simulink model "ADU_Integration_Y2016_simulation"  (R2016b)
settings: Solver=FixedStepDiscrete  StartTime=240  StopTime=300  FixedStep=0.01  RelTol=1e-3  EnableMultiTasking=on
PostLoadFcn:
  | , if any(exist('dsrtsu_mdlpostloadfcn', 'file') == [2, 3, 6]), try dsrtsu_mdlpostloadfcn('Execute', bdroot); catch fprintf('Error in PostLoadFcn (dsrtsu_mdlpostloadfcn) for model "%s":\n %s\n', bdroot, lasterr); end, end,
InitFcn:
  | load 'data/chi2_dat';
  | load 'data/innerLine_struct';
  | load 'data/middleLine_struct';
  | load 'data/outerLine_struct';
  | load 'data/innerLine';
  | load 'data/middleLine';
  | load 'data/outerLine';
  | load 'data/landmarks_patac_schimmel_ccw';
  | load 'data/patac_navi_array';
  | load 'data/sensor';
  | load 'data/map_struct';
  | addpath map_src
  | Integration_Parameter;
  | load 'TestData_001';
values from neighbouring files (symbols this model uses):
  TestData_001 =     [TestData_001.mat]
undefined symbols (not defined in the file or in its folder): a, chi2_dat, innerLine, landmarks_patac_schimmel_ccw, middleLine, outerLine, patac_navi_array, StartNum
libraries: simulink x36, rtican x1
(part 4 of 20)

== system ADU_Integration_Y2016_simulation/LogData/Sensor_ESR/Data_13 ==
  1-D Lookup Table1 : Lookup_n-D  NumberOfTableDimensions=1  BreakpointsForDimension1=TestData_001.X.Data  Table=TestData_001.Y(206+4*a).Data  RndMeth=Simplest  InputSameDT=on
  1-D Lookup Table2 : Lookup_n-D  NumberOfTableDimensions=1  BreakpointsForDimension1=TestData_001.X.Data  Table=TestData_001.Y(205+4*a).Data  RndMeth=Simplest  InputSameDT=on
  1-D Lookup Table3 : Lookup_n-D  NumberOfTableDimensions=1  BreakpointsForDimension1=TestData_001.X.Data  Table=TestData_001.Y(207+4*a).Data  RndMeth=Simplest  InputSameDT=on
  1-D Lookup Table4 : Lookup_n-D  NumberOfTableDimensions=1  BreakpointsForDimension1=TestData_001.X.Data  Table=TestData_001.Y(208+4*a).Data  RndMeth=Simplest  InputSameDT=on
  Mux5 : Mux
  Quantizer9 : Quantizer  QuantizationInterval=1
  Out1 : Outport
  wires:
  Mux5/1 -> Out1/1
  [Clock] -> 1-D Lookup Table2/1, 1-D Lookup Table4/1, 1-D Lookup Table3/1, 1-D Lookup Table1/1
  1-D Lookup Table4/1 -> Mux5/4
  Quantizer9/1 -> Mux5/1
  1-D Lookup Table2/1 -> Quantizer9/1
  1-D Lookup Table1/1 -> Mux5/2  "Data"
  1-D Lookup Table3/1 -> Mux5/3

== system ADU_Integration_Y2016_simulation/LogData/Sensor_ESR/Data_14 ==
  1-D Lookup Table1 : Lookup_n-D  NumberOfTableDimensions=1  BreakpointsForDimension1=TestData_001.X.Data  Table=TestData_001.Y(206+4*a).Data  RndMeth=Simplest  InputSameDT=on
  1-D Lookup Table2 : Lookup_n-D  NumberOfTableDimensions=1  BreakpointsForDimension1=TestData_001.X.Data  Table=TestData_001.Y(205+4*a).Data  RndMeth=Simplest  InputSameDT=on
  1-D Lookup Table3 : Lookup_n-D  NumberOfTableDimensions=1  BreakpointsForDimension1=TestData_001.X.Data  Table=TestData_001.Y(207+4*a).Data  RndMeth=Simplest  InputSameDT=on
  1-D Lookup Table4 : Lookup_n-D  NumberOfTableDimensions=1  BreakpointsForDimension1=TestData_001.X.Data  Table=TestData_001.Y(208+4*a).Data  RndMeth=Simplest  InputSameDT=on
  Mux5 : Mux
  Quantizer9 : Quantizer  QuantizationInterval=1
  Out1 : Outport
  wires:
  1-D Lookup Table3/1 -> Mux5/3
  1-D Lookup Table1/1 -> Mux5/2  "Data"
  1-D Lookup Table2/1 -> Quantizer9/1
  Quantizer9/1 -> Mux5/1
  1-D Lookup Table4/1 -> Mux5/4
  [Clock] -> 1-D Lookup Table1/1, 1-D Lookup Table3/1, 1-D Lookup Table4/1, 1-D Lookup Table2/1
  Mux5/1 -> Out1/1

== system ADU_Integration_Y2016_simulation/LogData/Sensor_ESR/Data_15 ==
  1-D Lookup Table1 : Lookup_n-D  NumberOfTableDimensions=1  BreakpointsForDimension1=TestData_001.X.Data  Table=TestData_001.Y(206+4*a).Data  RndMeth=Simplest  InputSameDT=on
  1-D Lookup Table2 : Lookup_n-D  NumberOfTableDimensions=1  BreakpointsForDimension1=TestData_001.X.Data  Table=TestData_001.Y(205+4*a).Data  RndMeth=Simplest  InputSameDT=on
  1-D Lookup Table3 : Lookup_n-D  NumberOfTableDimensions=1  BreakpointsForDimension1=TestData_001.X.Data  Table=TestData_001.Y(207+4*a).Data  RndMeth=Simplest  InputSameDT=on
  1-D Lookup Table4 : Lookup_n-D  NumberOfTableDimensions=1  BreakpointsForDimension1=TestData_001.X.Data  Table=TestData_001.Y(208+4*a).Data  RndMeth=Simplest  InputSameDT=on
  Mux5 : Mux
  Quantizer9 : Quantizer  QuantizationInterval=1
  Out1 : Outport
  wires:
  Mux5/1 -> Out1/1
  [Clock] -> 1-D Lookup Table2/1, 1-D Lookup Table4/1, 1-D Lookup Table3/1, 1-D Lookup Table1/1
  1-D Lookup Table4/1 -> Mux5/4
  Quantizer9/1 -> Mux5/1
  1-D Lookup Table2/1 -> Quantizer9/1
  1-D Lookup Table1/1 -> Mux5/2  "Data"
  1-D Lookup Table3/1 -> Mux5/3

== system ADU_Integration_Y2016_simulation/LogData/Sensor_ESR/Data_16 ==
  1-D Lookup Table1 : Lookup_n-D  NumberOfTableDimensions=1  BreakpointsForDimension1=TestData_001.X.Data  Table=TestData_001.Y(206+4*a).Data  RndMeth=Simplest  InputSameDT=on
  1-D Lookup Table2 : Lookup_n-D  NumberOfTableDimensions=1  BreakpointsForDimension1=TestData_001.X.Data  Table=TestData_001.Y(205+4*a).Data  RndMeth=Simplest  InputSameDT=on
  1-D Lookup Table3 : Lookup_n-D  NumberOfTableDimensions=1  BreakpointsForDimension1=TestData_001.X.Data  Table=TestData_001.Y(207+4*a).Data  RndMeth=Simplest  InputSameDT=on
  1-D Lookup Table4 : Lookup_n-D  NumberOfTableDimensions=1  BreakpointsForDimension1=TestData_001.X.Data  Table=TestData_001.Y(208+4*a).Data  RndMeth=Simplest  InputSameDT=on
  Mux5 : Mux
  Quantizer9 : Quantizer  QuantizationInterval=1
  Out1 : Outport
  wires:
  1-D Lookup Table3/1 -> Mux5/3
  1-D Lookup Table1/1 -> Mux5/2  "Data"
  1-D Lookup Table2/1 -> Quantizer9/1
  Quantizer9/1 -> Mux5/1
  1-D Lookup Table4/1 -> Mux5/4
  [Clock] -> 1-D Lookup Table1/1, 1-D Lookup Table3/1, 1-D Lookup Table4/1, 1-D Lookup Table2/1
  Mux5/1 -> Out1/1

== system ADU_Integration_Y2016_simulation/LogData/Sensor_ESR/Data_17 ==
  1-D Lookup Table1 : Lookup_n-D  NumberOfTableDimensions=1  BreakpointsForDimension1=TestData_001.X.Data  Table=TestData_001.Y(206+4*a).Data  RndMeth=Simplest  InputSameDT=on
  1-D Lookup Table2 : Lookup_n-D  NumberOfTableDimensions=1  BreakpointsForDimension1=TestData_001.X.Data  Table=TestData_001.Y(205+4*a).Data  RndMeth=Simplest  InputSameDT=on
  1-D Lookup Table3 : Lookup_n-D  NumberOfTableDimensions=1  BreakpointsForDimension1=TestData_001.X.Data  Table=TestData_001.Y(207+4*a).Data  RndMeth=Simplest  InputSameDT=on
  1-D Lookup Table4 : Lookup_n-D  NumberOfTableDimensions=1  BreakpointsForDimension1=TestData_001.X.Data  Table=TestData_001.Y(208+4*a).Data  RndMeth=Simplest  InputSameDT=on
  Mux5 : Mux
  Quantizer9 : Quantizer  QuantizationInterval=1
  Out1 : Outport
  wires:
  Mux5/1 -> Out1/1
  [Clock] -> 1-D Lookup Table2/1, 1-D Lookup Table4/1, 1-D Lookup Table3/1, 1-D Lookup Table1/1
  1-D Lookup Table4/1 -> Mux5/4
  Quantizer9/1 -> Mux5/1
  1-D Lookup Table2/1 -> Quantizer9/1
  1-D Lookup Table1/1 -> Mux5/2  "Data"
  1-D Lookup Table3/1 -> Mux5/3

== system ADU_Integration_Y2016_simulation/LogData/Sensor_ESR/Data_18 ==
  1-D Lookup Table1 : Lookup_n-D  NumberOfTableDimensions=1  BreakpointsForDimension1=TestData_001.X.Data  Table=TestData_001.Y(206+4*a).Data  RndMeth=Simplest  InputSameDT=on
  1-D Lookup Table2 : Lookup_n-D  NumberOfTableDimensions=1  BreakpointsForDimension1=TestData_001.X.Data  Table=TestData_001.Y(205+4*a).Data  RndMeth=Simplest  InputSameDT=on
  1-D Lookup Table3 : Lookup_n-D  NumberOfTableDimensions=1  BreakpointsForDimension1=TestData_001.X.Data  Table=TestData_001.Y(207+4*a).Data  RndMeth=Simplest  InputSameDT=on
  1-D Lookup Table4 : Lookup_n-D  NumberOfTableDimensions=1  BreakpointsForDimension1=TestData_001.X.Data  Table=TestData_001.Y(208+4*a).Data  RndMeth=Simplest  InputSameDT=on
  Mux5 : Mux
  Quantizer9 : Quantizer  QuantizationInterval=1
  Out1 : Outport
  wires:
  1-D Lookup Table3/1 -> Mux5/3
  1-D Lookup Table1/1 -> Mux5/2  "Data"
  1-D Lookup Table2/1 -> Quantizer9/1
  Quantizer9/1 -> Mux5/1
  1-D Lookup Table4/1 -> Mux5/4
  [Clock] -> 1-D Lookup Table1/1, 1-D Lookup Table3/1, 1-D Lookup Table4/1, 1-D Lookup Table2/1
  Mux5/1 -> Out1/1

== system ADU_Integration_Y2016_simulation/LogData/Sensor_ESR/Data_19 ==
  1-D Lookup Table1 : Lookup_n-D  NumberOfTableDimensions=1  BreakpointsForDimension1=TestData_001.X.Data  Table=TestData_001.Y(206+4*a).Data  RndMeth=Simplest  InputSameDT=on
  1-D Lookup Table2 : Lookup_n-D  NumberOfTableDimensions=1  BreakpointsForDimension1=TestData_001.X.Data  Table=TestData_001.Y(205+4*a).Data  RndMeth=Simplest  InputSameDT=on
  1-D Lookup Table3 : Lookup_n-D  NumberOfTableDimensions=1  BreakpointsForDimension1=TestData_001.X.Data  Table=TestData_001.Y(207+4*a).Data  RndMeth=Simplest  InputSameDT=on
  1-D Lookup Table4 : Lookup_n-D  NumberOfTableDimensions=1  BreakpointsForDimension1=TestData_001.X.Data  Table=TestData_001.Y(208+4*a).Data  RndMeth=Simplest  InputSameDT=on
  Mux5 : Mux
  Quantizer9 : Quantizer  QuantizationInterval=1
  Out1 : Outport
  wires:
  Mux5/1 -> Out1/1
  [Clock] -> 1-D Lookup Table2/1, 1-D Lookup Table4/1, 1-D Lookup Table3/1, 1-D Lookup Table1/1
  1-D Lookup Table4/1 -> Mux5/4
  Quantizer9/1 -> Mux5/1
  1-D Lookup Table2/1 -> Quantizer9/1
  1-D Lookup Table1/1 -> Mux5/2  "Data"
  1-D Lookup Table3/1 -> Mux5/3

== system ADU_Integration_Y2016_simulation/LogData/Sensor_ESR/Data_2 ==
  1-D Lookup Table1 : Lookup_n-D  NumberOfTableDimensions=1  BreakpointsForDimension1=TestData_001.X.Data  Table=TestData_001.Y(206+4*a).Data  RndMeth=Simplest  InputSameDT=on
  1-D Lookup Table2 : Lookup_n-D  NumberOfTableDimensions=1  BreakpointsForDimension1=TestData_001.X.Data  Table=TestData_001.Y(205+4*a).Data  RndMeth=Simplest  InputSameDT=on
  1-D Lookup Table3 : Lookup_n-D  NumberOfTableDimensions=1  BreakpointsForDimension1=TestData_001.X.Data  Table=TestData_001.Y(207+4*a).Data  RndMeth=Simplest  InputSameDT=on
  1-D Lookup Table4 : Lookup_n-D  NumberOfTableDimensions=1  BreakpointsForDimension1=TestData_001.X.Data  Table=TestData_001.Y(208+4*a).Data  RndMeth=Simplest  InputSameDT=on
  Mux5 : Mux
  Quantizer9 : Quantizer  QuantizationInterval=1
  Out1 : Outport
  wires:
  1-D Lookup Table3/1 -> Mux5/3
  1-D Lookup Table1/1 -> Mux5/2  "Data"
  1-D Lookup Table2/1 -> Quantizer9/1
  Quantizer9/1 -> Mux5/1
  1-D Lookup Table4/1 -> Mux5/4
  [Clock] -> 1-D Lookup Table1/1, 1-D Lookup Table3/1, 1-D Lookup Table4/1, 1-D Lookup Table2/1
  Mux5/1 -> Out1/1

== system ADU_Integration_Y2016_simulation/LogData/Sensor_ESR/Data_20 ==
  1-D Lookup Table1 : Lookup_n-D  NumberOfTableDimensions=1  BreakpointsForDimension1=TestData_001.X.Data  Table=TestData_001.Y(206+4*a).Data  RndMeth=Simplest  InputSameDT=on
  1-D Lookup Table2 : Lookup_n-D  NumberOfTableDimensions=1  BreakpointsForDimension1=TestData_001.X.Data  Table=TestData_001.Y(205+4*a).Data  RndMeth=Simplest  InputSameDT=on
  1-D Lookup Table3 : Lookup_n-D  NumberOfTableDimensions=1  BreakpointsForDimension1=TestData_001.X.Data  Table=TestData_001.Y(207+4*a).Data  RndMeth=Simplest  InputSameDT=on
  1-D Lookup Table4 : Lookup_n-D  NumberOfTableDimensions=1  BreakpointsForDimension1=TestData_001.X.Data  Table=TestData_001.Y(208+4*a).Data  RndMeth=Simplest  InputSameDT=on
  Mux5 : Mux
  Quantizer9 : Quantizer  QuantizationInterval=1
  Out1 : Outport
  wires:
  1-D Lookup Table3/1 -> Mux5/3
  1-D Lookup Table1/1 -> Mux5/2  "Data"
  1-D Lookup Table2/1 -> Quantizer9/1
  Quantizer9/1 -> Mux5/1
  1-D Lookup Table4/1 -> Mux5/4
  [Clock] -> 1-D Lookup Table1/1, 1-D Lookup Table3/1, 1-D Lookup Table4/1, 1-D Lookup Table2/1
  Mux5/1 -> Out1/1

== system ADU_Integration_Y2016_simulation/LogData/Sensor_ESR/Data_21 ==
  1-D Lookup Table1 : Lookup_n-D  NumberOfTableDimensions=1  BreakpointsForDimension1=TestData_001.X.Data  Table=TestData_001.Y(206+4*a).Data  RndMeth=Simplest  InputSameDT=on
  1-D Lookup Table2 : Lookup_n-D  NumberOfTableDimensions=1  BreakpointsForDimension1=TestData_001.X.Data  Table=TestData_001.Y(205+4*a).Data  RndMeth=Simplest  InputSameDT=on
  1-D Lookup Table3 : Lookup_n-D  NumberOfTableDimensions=1  BreakpointsForDimension1=TestData_001.X.Data  Table=TestData_001.Y(207+4*a).Data  RndMeth=Simplest  InputSameDT=on
  1-D Lookup Table4 : Lookup_n-D  NumberOfTableDimensions=1  BreakpointsForDimension1=TestData_001.X.Data  Table=TestData_001.Y(208+4*a).Data  RndMeth=Simplest  InputSameDT=on
  Mux5 : Mux
  Quantizer9 : Quantizer  QuantizationInterval=1
  Out1 : Outport
  wires:
  Mux5/1 -> Out1/1
  [Clock] -> 1-D Lookup Table2/1, 1-D Lookup Table4/1, 1-D Lookup Table3/1, 1-D Lookup Table1/1
  1-D Lookup Table4/1 -> Mux5/4
  Quantizer9/1 -> Mux5/1
  1-D Lookup Table2/1 -> Quantizer9/1
  1-D Lookup Table1/1 -> Mux5/2  "Data"
  1-D Lookup Table3/1 -> Mux5/3

== system ADU_Integration_Y2016_simulation/LogData/Sensor_ESR/Data_22 ==
  1-D Lookup Table1 : Lookup_n-D  NumberOfTableDimensions=1  BreakpointsForDimension1=TestData_001.X.Data  Table=TestData_001.Y(206+4*a).Data  RndMeth=Simplest  InputSameDT=on
  1-D Lookup Table2 : Lookup_n-D  NumberOfTableDimensions=1  BreakpointsForDimension1=TestData_001.X.Data  Table=TestData_001.Y(205+4*a).Data  RndMeth=Simplest  InputSameDT=on
  1-D Lookup Table3 : Lookup_n-D  NumberOfTableDimensions=1  BreakpointsForDimension1=TestData_001.X.Data  Table=TestData_001.Y(207+4*a).Data  RndMeth=Simplest  InputSameDT=on
  1-D Lookup Table4 : Lookup_n-D  NumberOfTableDimensions=1  BreakpointsForDimension1=TestData_001.X.Data  Table=TestData_001.Y(208+4*a).Data  RndMeth=Simplest  InputSameDT=on
  Mux5 : Mux
  Quantizer9 : Quantizer  QuantizationInterval=1
  Out1 : Outport
  wires:
  1-D Lookup Table3/1 -> Mux5/3
  1-D Lookup Table1/1 -> Mux5/2  "Data"
  1-D Lookup Table2/1 -> Quantizer9/1
  Quantizer9/1 -> Mux5/1
  1-D Lookup Table4/1 -> Mux5/4
  [Clock] -> 1-D Lookup Table1/1, 1-D Lookup Table3/1, 1-D Lookup Table4/1, 1-D Lookup Table2/1
  Mux5/1 -> Out1/1

== system ADU_Integration_Y2016_simulation/LogData/Sensor_ESR/Data_23 ==
  1-D Lookup Table1 : Lookup_n-D  NumberOfTableDimensions=1  BreakpointsForDimension1=TestData_001.X.Data  Table=TestData_001.Y(206+4*a).Data  RndMeth=Simplest  InputSameDT=on
  1-D Lookup Table2 : Lookup_n-D  NumberOfTableDimensions=1  BreakpointsForDimension1=TestData_001.X.Data  Table=TestData_001.Y(205+4*a).Data  RndMeth=Simplest  InputSameDT=on
  1-D Lookup Table3 : Lookup_n-D  NumberOfTableDimensions=1  BreakpointsForDimension1=TestData_001.X.Data  Table=TestData_001.Y(207+4*a).Data  RndMeth=Simplest  InputSameDT=on
  1-D Lookup Table4 : Lookup_n-D  NumberOfTableDimensions=1  BreakpointsForDimension1=TestData_001.X.Data  Table=TestData_001.Y(208+4*a).Data  RndMeth=Simplest  InputSameDT=on
  Mux5 : Mux
  Quantizer9 : Quantizer  QuantizationInterval=1
  Out1 : Outport
  wires:
  Mux5/1 -> Out1/1
  [Clock] -> 1-D Lookup Table2/1, 1-D Lookup Table4/1, 1-D Lookup Table3/1, 1-D Lookup Table1/1
  1-D Lookup Table4/1 -> Mux5/4
  Quantizer9/1 -> Mux5/1
  1-D Lookup Table2/1 -> Quantizer9/1
  1-D Lookup Table1/1 -> Mux5/2  "Data"
  1-D Lookup Table3/1 -> Mux5/3

== system ADU_Integration_Y2016_simulation/LogData/Sensor_ESR/Data_24 ==
  1-D Lookup Table1 : Lookup_n-D  NumberOfTableDimensions=1  BreakpointsForDimension1=TestData_001.X.Data  Table=TestData_001.Y(206+4*a).Data  RndMeth=Simplest  InputSameDT=on
  1-D Lookup Table2 : Lookup_n-D  NumberOfTableDimensions=1  BreakpointsForDimension1=TestData_001.X.Data  Table=TestData_001.Y(205+4*a).Data  RndMeth=Simplest  InputSameDT=on
  1-D Lookup Table3 : Lookup_n-D  NumberOfTableDimensions=1  BreakpointsForDimension1=TestData_001.X.Data  Table=TestData_001.Y(207+4*a).Data  RndMeth=Simplest  InputSameDT=on
  1-D Lookup Table4 : Lookup_n-D  NumberOfTableDimensions=1  BreakpointsForDimension1=TestData_001.X.Data  Table=TestData_001.Y(208+4*a).Data  RndMeth=Simplest  InputSameDT=on
  Mux5 : Mux
  Quantizer9 : Quantizer  QuantizationInterval=1
  Out1 : Outport
  wires:
  1-D Lookup Table3/1 -> Mux5/3
  1-D Lookup Table1/1 -> Mux5/2  "Data"
  1-D Lookup Table2/1 -> Quantizer9/1
  Quantizer9/1 -> Mux5/1
  1-D Lookup Table4/1 -> Mux5/4
  [Clock] -> 1-D Lookup Table1/1, 1-D Lookup Table3/1, 1-D Lookup Table4/1, 1-D Lookup Table2/1
  Mux5/1 -> Out1/1

== system ADU_Integration_Y2016_simulation/LogData/Sensor_ESR/Data_25 ==
  1-D Lookup Table1 : Lookup_n-D  NumberOfTableDimensions=1  BreakpointsForDimension1=TestData_001.X.Data  Table=TestData_001.Y(206+4*a).Data  RndMeth=Simplest  InputSameDT=on
  1-D Lookup Table2 : Lookup_n-D  NumberOfTableDimensions=1  BreakpointsForDimension1=TestData_001.X.Data  Table=TestData_001.Y(205+4*a).Data  RndMeth=Simplest  InputSameDT=on
  1-D Lookup Table3 : Lookup_n-D  NumberOfTableDimensions=1  BreakpointsForDimension1=TestData_001.X.Data  Table=TestData_001.Y(207+4*a).Data  RndMeth=Simplest  InputSameDT=on
  1-D Lookup Table4 : Lookup_n-D  NumberOfTableDimensions=1  BreakpointsForDimension1=TestData_001.X.Data  Table=TestData_001.Y(208+4*a).Data  RndMeth=Simplest  InputSameDT=on
  Mux5 : Mux
  Quantizer9 : Quantizer  QuantizationInterval=1
  Out1 : Outport
  wires:
  Mux5/1 -> Out1/1
  [Clock] -> 1-D Lookup Table2/1, 1-D Lookup Table4/1, 1-D Lookup Table3/1, 1-D Lookup Table1/1
  1-D Lookup Table4/1 -> Mux5/4
  Quantizer9/1 -> Mux5/1
  1-D Lookup Table2/1 -> Quantizer9/1
  1-D Lookup Table1/1 -> Mux5/2  "Data"
  1-D Lookup Table3/1 -> Mux5/3

== system ADU_Integration_Y2016_simulation/LogData/Sensor_ESR/Data_26 ==
  1-D Lookup Table1 : Lookup_n-D  NumberOfTableDimensions=1  BreakpointsForDimension1=TestData_001.X.Data  Table=TestData_001.Y(206+4*a).Data  RndMeth=Simplest  InputSameDT=on
  1-D Lookup Table2 : Lookup_n-D  NumberOfTableDimensions=1  BreakpointsForDimension1=TestData_001.X.Data  Table=TestData_001.Y(205+4*a).Data  RndMeth=Simplest  InputSameDT=on
  1-D Lookup Table3 : Lookup_n-D  NumberOfTableDimensions=1  BreakpointsForDimension1=TestData_001.X.Data  Table=TestData_001.Y(207+4*a).Data  RndMeth=Simplest  InputSameDT=on
  1-D Lookup Table4 : Lookup_n-D  NumberOfTableDimensions=1  BreakpointsForDimension1=TestData_001.X.Data  Table=TestData_001.Y(208+4*a).Data  RndMeth=Simplest  InputSameDT=on
  Mux5 : Mux
  Quantizer9 : Quantizer  QuantizationInterval=1
  Out1 : Outport
  wires:
  1-D Lookup Table3/1 -> Mux5/3
  1-D Lookup Table1/1 -> Mux5/2  "Data"
  1-D Lookup Table2/1 -> Quantizer9/1
  Quantizer9/1 -> Mux5/1
  1-D Lookup Table4/1 -> Mux5/4
  [Clock] -> 1-D Lookup Table1/1, 1-D Lookup Table3/1, 1-D Lookup Table4/1, 1-D Lookup Table2/1
  Mux5/1 -> Out1/1

== system ADU_Integration_Y2016_simulation/LogData/Sensor_ESR/Data_27 ==
  1-D Lookup Table1 : Lookup_n-D  NumberOfTableDimensions=1  BreakpointsForDimension1=TestData_001.X.Data  Table=TestData_001.Y(206+4*a).Data  RndMeth=Simplest  InputSameDT=on
  1-D Lookup Table2 : Lookup_n-D  NumberOfTableDimensions=1  BreakpointsForDimension1=TestData_001.X.Data  Table=TestData_001.Y(205+4*a).Data  RndMeth=Simplest  InputSameDT=on
  1-D Lookup Table3 : Lookup_n-D  NumberOfTableDimensions=1  BreakpointsForDimension1=TestData_001.X.Data  Table=TestData_001.Y(207+4*a).Data  RndMeth=Simplest  InputSameDT=on
  1-D Lookup Table4 : Lookup_n-D  NumberOfTableDimensions=1  BreakpointsForDimension1=TestData_001.X.Data  Table=TestData_001.Y(208+4*a).Data  RndMeth=Simplest  InputSameDT=on
  Mux5 : Mux
  Quantizer9 : Quantizer  QuantizationInterval=1
  Out1 : Outport
  wires:
  Mux5/1 -> Out1/1
  [Clock] -> 1-D Lookup Table2/1, 1-D Lookup Table4/1, 1-D Lookup Table3/1, 1-D Lookup Table1/1
  1-D Lookup Table4/1 -> Mux5/4
  Quantizer9/1 -> Mux5/1
  1-D Lookup Table2/1 -> Quantizer9/1
  1-D Lookup Table1/1 -> Mux5/2  "Data"
  1-D Lookup Table3/1 -> Mux5/3

== system ADU_Integration_Y2016_simulation/LogData/Sensor_ESR/Data_28 ==
  1-D Lookup Table1 : Lookup_n-D  NumberOfTableDimensions=1  BreakpointsForDimension1=TestData_001.X.Data  Table=TestData_001.Y(206+4*a).Data  RndMeth=Simplest  InputSameDT=on
  1-D Lookup Table2 : Lookup_n-D  NumberOfTableDimensions=1  BreakpointsForDimension1=TestData_001.X.Data  Table=TestData_001.Y(205+4*a).Data  RndMeth=Simplest  InputSameDT=on
  1-D Lookup Table3 : Lookup_n-D  NumberOfTableDimensions=1  BreakpointsForDimension1=TestData_001.X.Data  Table=TestData_001.Y(207+4*a).Data  RndMeth=Simplest  InputSameDT=on
  1-D Lookup Table4 : Lookup_n-D  NumberOfTableDimensions=1  BreakpointsForDimension1=TestData_001.X.Data  Table=TestData_001.Y(208+4*a).Data  RndMeth=Simplest  InputSameDT=on
  Mux5 : Mux
  Quantizer9 : Quantizer  QuantizationInterval=1
  Out1 : Outport
  wires:
  1-D Lookup Table3/1 -> Mux5/3
  1-D Lookup Table1/1 -> Mux5/2  "Data"
  1-D Lookup Table2/1 -> Quantizer9/1
  Quantizer9/1 -> Mux5/1
  1-D Lookup Table4/1 -> Mux5/4
  [Clock] -> 1-D Lookup Table1/1, 1-D Lookup Table3/1, 1-D Lookup Table4/1, 1-D Lookup Table2/1
  Mux5/1 -> Out1/1

== system ADU_Integration_Y2016_simulation/LogData/Sensor_ESR/Data_29 ==
  1-D Lookup Table1 : Lookup_n-D  NumberOfTableDimensions=1  BreakpointsForDimension1=TestData_001.X.Data  Table=TestData_001.Y(206+4*a).Data  RndMeth=Simplest  InputSameDT=on
  1-D Lookup Table2 : Lookup_n-D  NumberOfTableDimensions=1  BreakpointsForDimension1=TestData_001.X.Data  Table=TestData_001.Y(205+4*a).Data  RndMeth=Simplest  InputSameDT=on
  1-D Lookup Table3 : Lookup_n-D  NumberOfTableDimensions=1  BreakpointsForDimension1=TestData_001.X.Data  Table=TestData_001.Y(207+4*a).Data  RndMeth=Simplest  InputSameDT=on
  1-D Lookup Table4 : Lookup_n-D  NumberOfTableDimensions=1  BreakpointsForDimension1=TestData_001.X.Data  Table=TestData_001.Y(208+4*a).Data  RndMeth=Simplest  InputSameDT=on
  Mux5 : Mux
  Quantizer9 : Quantizer  QuantizationInterval=1
  Out1 : Outport
  wires:
  Mux5/1 -> Out1/1
  [Clock] -> 1-D Lookup Table2/1, 1-D Lookup Table4/1, 1-D Lookup Table3/1, 1-D Lookup Table1/1
  1-D Lookup Table4/1 -> Mux5/4
  Quantizer9/1 -> Mux5/1
  1-D Lookup Table2/1 -> Quantizer9/1
  1-D Lookup Table1/1 -> Mux5/2  "Data"
  1-D Lookup Table3/1 -> Mux5/3

== system ADU_Integration_Y2016_simulation/LogData/Sensor_ESR/Data_3 ==
  1-D Lookup Table1 : Lookup_n-D  NumberOfTableDimensions=1  BreakpointsForDimension1=TestData_001.X.Data  Table=TestData_001.Y(206+4*a).Data  RndMeth=Simplest  InputSameDT=on
  1-D Lookup Table2 : Lookup_n-D  NumberOfTableDimensions=1  BreakpointsForDimension1=TestData_001.X.Data  Table=TestData_001.Y(205+4*a).Data  RndMeth=Simplest  InputSameDT=on
  1-D Lookup Table3 : Lookup_n-D  NumberOfTableDimensions=1  BreakpointsForDimension1=TestData_001.X.Data  Table=TestData_001.Y(207+4*a).Data  RndMeth=Simplest  InputSameDT=on
  1-D Lookup Table4 : Lookup_n-D  NumberOfTableDimensions=1  BreakpointsForDimension1=TestData_001.X.Data  Table=TestData_001.Y(208+4*a).Data  RndMeth=Simplest  InputSameDT=on
  Mux5 : Mux
  Quantizer9 : Quantizer  QuantizationInterval=1
  Out1 : Outport
  wires:
  Mux5/1 -> Out1/1
  [Clock] -> 1-D Lookup Table2/1, 1-D Lookup Table4/1, 1-D Lookup Table3/1, 1-D Lookup Table1/1
  1-D Lookup Table4/1 -> Mux5/4
  Quantizer9/1 -> Mux5/1
  1-D Lookup Table2/1 -> Quantizer9/1
  1-D Lookup Table1/1 -> Mux5/2  "Data"
  1-D Lookup Table3/1 -> Mux5/3

== system ADU_Integration_Y2016_simulation/LogData/Sensor_ESR/Data_30 ==
  1-D Lookup Table1 : Lookup_n-D  NumberOfTableDimensions=1  BreakpointsForDimension1=TestData_001.X.Data  Table=TestData_001.Y(206+4*a).Data  RndMeth=Simplest  InputSameDT=on
  1-D Lookup Table2 : Lookup_n-D  NumberOfTableDimensions=1  BreakpointsForDimension1=TestData_001.X.Data  Table=TestData_001.Y(205+4*a).Data  RndMeth=Simplest  InputSameDT=on
  1-D Lookup Table3 : Lookup_n-D  NumberOfTableDimensions=1  BreakpointsForDimension1=TestData_001.X.Data  Table=TestData_001.Y(207+4*a).Data  RndMeth=Simplest  InputSameDT=on
  1-D Lookup Table4 : Lookup_n-D  NumberOfTableDimensions=1  BreakpointsForDimension1=TestData_001.X.Data  Table=TestData_001.Y(208+4*a).Data  RndMeth=Simplest  InputSameDT=on
  Mux5 : Mux
  Quantizer9 : Quantizer  QuantizationInterval=1
  Out1 : Outport
  wires:
  1-D Lookup Table3/1 -> Mux5/3
  1-D Lookup Table1/1 -> Mux5/2  "Data"
  1-D Lookup Table2/1 -> Quantizer9/1
  Quantizer9/1 -> Mux5/1
  1-D Lookup Table4/1 -> Mux5/4
  [Clock] -> 1-D Lookup Table1/1, 1-D Lookup Table3/1, 1-D Lookup Table4/1, 1-D Lookup Table2/1
  Mux5/1 -> Out1/1

== system ADU_Integration_Y2016_simulation/LogData/Sensor_ESR/Data_31 ==
  1-D Lookup Table1 : Lookup_n-D  NumberOfTableDimensions=1  BreakpointsForDimension1=TestData_001.X.Data  Table=TestData_001.Y(206+4*a).Data  RndMeth=Simplest  InputSameDT=on
  1-D Lookup Table2 : Lookup_n-D  NumberOfTableDimensions=1  BreakpointsForDimension1=TestData_001.X.Data  Table=TestData_001.Y(205+4*a).Data  RndMeth=Simplest  InputSameDT=on
  1-D Lookup Table3 : Lookup_n-D  NumberOfTableDimensions=1  BreakpointsForDimension1=TestData_001.X.Data  Table=TestData_001.Y(207+4*a).Data  RndMeth=Simplest  InputSameDT=on
  1-D Lookup Table4 : Lookup_n-D  NumberOfTableDimensions=1  BreakpointsForDimension1=TestData_001.X.Data  Table=TestData_001.Y(208+4*a).Data  RndMeth=Simplest  InputSameDT=on
  Mux5 : Mux
  Quantizer9 : Quantizer  QuantizationInterval=1
  Out1 : Outport
  wires:
  Mux5/1 -> Out1/1
  [Clock] -> 1-D Lookup Table2/1, 1-D Lookup Table4/1, 1-D Lookup Table3/1, 1-D Lookup Table1/1
  1-D Lookup Table4/1 -> Mux5/4
  Quantizer9/1 -> Mux5/1
  1-D Lookup Table2/1 -> Quantizer9/1
  1-D Lookup Table1/1 -> Mux5/2  "Data"
  1-D Lookup Table3/1 -> Mux5/3

== system ADU_Integration_Y2016_simulation/LogData/Sensor_ESR/Data_32 ==
  1-D Lookup Table1 : Lookup_n-D  NumberOfTableDimensions=1  BreakpointsForDimension1=TestData_001.X.Data  Table=TestData_001.Y(206+4*a).Data  RndMeth=Simplest  InputSameDT=on
  1-D Lookup Table2 : Lookup_n-D  NumberOfTableDimensions=1  BreakpointsForDimension1=TestData_001.X.Data  Table=TestData_001.Y(205+4*a).Data  RndMeth=Simplest  InputSameDT=on
  1-D Lookup Table3 : Lookup_n-D  NumberOfTableDimensions=1  BreakpointsForDimension1=TestData_001.X.Data  Table=TestData_001.Y(207+4*a).Data  RndMeth=Simplest  InputSameDT=on
  1-D Lookup Table4 : Lookup_n-D  NumberOfTableDimensions=1  BreakpointsForDimension1=TestData_001.X.Data  Table=TestData_001.Y(208+4*a).Data  RndMeth=Simplest  InputSameDT=on
  Mux5 : Mux
  Quantizer9 : Quantizer  QuantizationInterval=1
  Out1 : Outport
  wires:
  1-D Lookup Table3/1 -> Mux5/3
  1-D Lookup Table1/1 -> Mux5/2  "Data"
  1-D Lookup Table2/1 -> Quantizer9/1
  Quantizer9/1 -> Mux5/1
  1-D Lookup Table4/1 -> Mux5/4
  [Clock] -> 1-D Lookup Table1/1, 1-D Lookup Table3/1, 1-D Lookup Table4/1, 1-D Lookup Table2/1
  Mux5/1 -> Out1/1

== system ADU_Integration_Y2016_simulation/LogData/Sensor_ESR/Data_33 ==
  1-D Lookup Table1 : Lookup_n-D  NumberOfTableDimensions=1  BreakpointsForDimension1=TestData_001.X.Data  Table=TestData_001.Y(206+4*a).Data  RndMeth=Simplest  InputSameDT=on
  1-D Lookup Table2 : Lookup_n-D  NumberOfTableDimensions=1  BreakpointsForDimension1=TestData_001.X.Data  Table=TestData_001.Y(205+4*a).Data  RndMeth=Simplest  InputSameDT=on
  1-D Lookup Table3 : Lookup_n-D  NumberOfTableDimensions=1  BreakpointsForDimension1=TestData_001.X.Data  Table=TestData_001.Y(207+4*a).Data  RndMeth=Simplest  InputSameDT=on
  1-D Lookup Table4 : Lookup_n-D  NumberOfTableDimensions=1  BreakpointsForDimension1=TestData_001.X.Data  Table=TestData_001.Y(208+4*a).Data  RndMeth=Simplest  InputSameDT=on
  Mux5 : Mux
  Quantizer9 : Quantizer  QuantizationInterval=1
  Out1 : Outport
  wires:
  Mux5/1 -> Out1/1
  [Clock] -> 1-D Lookup Table2/1, 1-D Lookup Table4/1, 1-D Lookup Table3/1, 1-D Lookup Table1/1
  1-D Lookup Table4/1 -> Mux5/4
  Quantizer9/1 -> Mux5/1
  1-D Lookup Table2/1 -> Quantizer9/1
  1-D Lookup Table1/1 -> Mux5/2  "Data"
  1-D Lookup Table3/1 -> Mux5/3

== system ADU_Integration_Y2016_simulation/LogData/Sensor_ESR/Data_34 ==
  1-D Lookup Table1 : Lookup_n-D  NumberOfTableDimensions=1  BreakpointsForDimension1=TestData_001.X.Data  Table=TestData_001.Y(206+4*a).Data  RndMeth=Simplest  InputSameDT=on
  1-D Lookup Table2 : Lookup_n-D  NumberOfTableDimensions=1  BreakpointsForDimension1=TestData_001.X.Data  Table=TestData_001.Y(205+4*a).Data  RndMeth=Simplest  InputSameDT=on
  1-D Lookup Table3 : Lookup_n-D  NumberOfTableDimensions=1  BreakpointsForDimension1=TestData_001.X.Data  Table=TestData_001.Y(207+4*a).Data  RndMeth=Simplest  InputSameDT=on
  1-D Lookup Table4 : Lookup_n-D  NumberOfTableDimensions=1  BreakpointsForDimension1=TestData_001.X.Data  Table=TestData_001.Y(208+4*a).Data  RndMeth=Simplest  InputSameDT=on
  Mux5 : Mux
  Quantizer9 : Quantizer  QuantizationInterval=1
  Out1 : Outport
  wires:
  1-D Lookup Table3/1 -> Mux5/3
  1-D Lookup Table1/1 -> Mux5/2  "Data"
  1-D Lookup Table2/1 -> Quantizer9/1
  Quantizer9/1 -> Mux5/1
  1-D Lookup Table4/1 -> Mux5/4
  [Clock] -> 1-D Lookup Table1/1, 1-D Lookup Table3/1, 1-D Lookup Table4/1, 1-D Lookup Table2/1
  Mux5/1 -> Out1/1

== system ADU_Integration_Y2016_simulation/LogData/Sensor_ESR/Data_35 ==
  1-D Lookup Table1 : Lookup_n-D  NumberOfTableDimensions=1  BreakpointsForDimension1=TestData_001.X.Data  Table=TestData_001.Y(206+4*a).Data  RndMeth=Simplest  InputSameDT=on
  1-D Lookup Table2 : Lookup_n-D  NumberOfTableDimensions=1  BreakpointsForDimension1=TestData_001.X.Data  Table=TestData_001.Y(205+4*a).Data  RndMeth=Simplest  InputSameDT=on
  1-D Lookup Table3 : Lookup_n-D  NumberOfTableDimensions=1  BreakpointsForDimension1=TestData_001.X.Data  Table=TestData_001.Y(207+4*a).Data  RndMeth=Simplest  InputSameDT=on
  1-D Lookup Table4 : Lookup_n-D  NumberOfTableDimensions=1  BreakpointsForDimension1=TestData_001.X.Data  Table=TestData_001.Y(208+4*a).Data  RndMeth=Simplest  InputSameDT=on
  Mux5 : Mux
  Quantizer9 : Quantizer  QuantizationInterval=1
  Out1 : Outport
  wires:
  Mux5/1 -> Out1/1
  [Clock] -> 1-D Lookup Table2/1, 1-D Lookup Table4/1, 1-D Lookup Table3/1, 1-D Lookup Table1/1
  1-D Lookup Table4/1 -> Mux5/4
  Quantizer9/1 -> Mux5/1
  1-D Lookup Table2/1 -> Quantizer9/1
  1-D Lookup Table1/1 -> Mux5/2  "Data"
  1-D Lookup Table3/1 -> Mux5/3

== system ADU_Integration_Y2016_simulation/LogData/Sensor_ESR/Data_36 ==
  1-D Lookup Table1 : Lookup_n-D  NumberOfTableDimensions=1  BreakpointsForDimension1=TestData_001.X.Data  Table=TestData_001.Y(206+4*a).Data  RndMeth=Simplest  InputSameDT=on
  1-D Lookup Table2 : Lookup_n-D  NumberOfTableDimensions=1  BreakpointsForDimension1=TestData_001.X.Data  Table=TestData_001.Y(205+4*a).Data  RndMeth=Simplest  InputSameDT=on
  1-D Lookup Table3 : Lookup_n-D  NumberOfTableDimensions=1  BreakpointsForDimension1=TestData_001.X.Data  Table=TestData_001.Y(207+4*a).Data  RndMeth=Simplest  InputSameDT=on
  1-D Lookup Table4 : Lookup_n-D  NumberOfTableDimensions=1  BreakpointsForDimension1=TestData_001.X.Data  Table=TestData_001.Y(208+4*a).Data  RndMeth=Simplest  InputSameDT=on
  Mux5 : Mux
  Quantizer9 : Quantizer  QuantizationInterval=1
  Out1 : Outport
  wires:
  1-D Lookup Table3/1 -> Mux5/3
  1-D Lookup Table1/1 -> Mux5/2  "Data"
  1-D Lookup Table2/1 -> Quantizer9/1
  Quantizer9/1 -> Mux5/1
  1-D Lookup Table4/1 -> Mux5/4
  [Clock] -> 1-D Lookup Table1/1, 1-D Lookup Table3/1, 1-D Lookup Table4/1, 1-D Lookup Table2/1
  Mux5/1 -> Out1/1

== system ADU_Integration_Y2016_simulation/LogData/Sensor_ESR/Data_37 ==
  1-D Lookup Table1 : Lookup_n-D  NumberOfTableDimensions=1  BreakpointsForDimension1=TestData_001.X.Data  Table=TestData_001.Y(206+4*a).Data  RndMeth=Simplest  InputSameDT=on
  1-D Lookup Table2 : Lookup_n-D  NumberOfTableDimensions=1  BreakpointsForDimension1=TestData_001.X.Data  Table=TestData_001.Y(205+4*a).Data  RndMeth=Simplest  InputSameDT=on
  1-D Lookup Table3 : Lookup_n-D  NumberOfTableDimensions=1  BreakpointsForDimension1=TestData_001.X.Data  Table=TestData_001.Y(207+4*a).Data  RndMeth=Simplest  InputSameDT=on
  1-D Lookup Table4 : Lookup_n-D  NumberOfTableDimensions=1  BreakpointsForDimension1=TestData_001.X.Data  Table=TestData_001.Y(208+4*a).Data  RndMeth=Simplest  InputSameDT=on
  Mux5 : Mux
  Quantizer9 : Quantizer  QuantizationInterval=1
  Out1 : Outport
  wires:
  Mux5/1 -> Out1/1
  [Clock] -> 1-D Lookup Table2/1, 1-D Lookup Table4/1, 1-D Lookup Table3/1, 1-D Lookup Table1/1
  1-D Lookup Table4/1 -> Mux5/4
  Quantizer9/1 -> Mux5/1
  1-D Lookup Table2/1 -> Quantizer9/1
  1-D Lookup Table1/1 -> Mux5/2  "Data"
  1-D Lookup Table3/1 -> Mux5/3

== system ADU_Integration_Y2016_simulation/LogData/Sensor_ESR/Data_38 ==
  1-D Lookup Table1 : Lookup_n-D  NumberOfTableDimensions=1  BreakpointsForDimension1=TestData_001.X.Data  Table=TestData_001.Y(206+4*a).Data  RndMeth=Simplest  InputSameDT=on
  1-D Lookup Table2 : Lookup_n-D  NumberOfTableDimensions=1  BreakpointsForDimension1=TestData_001.X.Data  Table=TestData_001.Y(205+4*a).Data  RndMeth=Simplest  InputSameDT=on
  1-D Lookup Table3 : Lookup_n-D  NumberOfTableDimensions=1  BreakpointsForDimension1=TestData_001.X.Data  Table=TestData_001.Y(207+4*a).Data  RndMeth=Simplest  InputSameDT=on
  1-D Lookup Table4 : Lookup_n-D  NumberOfTableDimensions=1  BreakpointsForDimension1=TestData_001.X.Data  Table=TestData_001.Y(208+4*a).Data  RndMeth=Simplest  InputSameDT=on
  Mux5 : Mux
  Quantizer9 : Quantizer  QuantizationInterval=1
  Out1 : Outport
  wires:
  1-D Lookup Table3/1 -> Mux5/3
  1-D Lookup Table1/1 -> Mux5/2  "Data"
  1-D Lookup Table2/1 -> Quantizer9/1
  Quantizer9/1 -> Mux5/1
  1-D Lookup Table4/1 -> Mux5/4
  [Clock] -> 1-D Lookup Table1/1, 1-D Lookup Table3/1, 1-D Lookup Table4/1, 1-D Lookup Table2/1
  Mux5/1 -> Out1/1

== system ADU_Integration_Y2016_simulation/LogData/Sensor_ESR/Data_39 ==
  1-D Lookup Table1 : Lookup_n-D  NumberOfTableDimensions=1  BreakpointsForDimension1=TestData_001.X.Data  Table=TestData_001.Y(206+4*a).Data  RndMeth=Simplest  InputSameDT=on
  1-D Lookup Table2 : Lookup_n-D  NumberOfTableDimensions=1  BreakpointsForDimension1=TestData_001.X.Data  Table=TestData_001.Y(205+4*a).Data  RndMeth=Simplest  InputSameDT=on
  1-D Lookup Table3 : Lookup_n-D  NumberOfTableDimensions=1  BreakpointsForDimension1=TestData_001.X.Data  Table=TestData_001.Y(207+4*a).Data  RndMeth=Simplest  InputSameDT=on
  1-D Lookup Table4 : Lookup_n-D  NumberOfTableDimensions=1  BreakpointsForDimension1=TestData_001.X.Data  Table=TestData_001.Y(208+4*a).Data  RndMeth=Simplest  InputSameDT=on
  Mux5 : Mux
  Quantizer9 : Quantizer  QuantizationInterval=1
  Out1 : Outport
  wires:
  Mux5/1 -> Out1/1
  [Clock] -> 1-D Lookup Table2/1, 1-D Lookup Table4/1, 1-D Lookup Table3/1, 1-D Lookup Table1/1
  1-D Lookup Table4/1 -> Mux5/4
  Quantizer9/1 -> Mux5/1
  1-D Lookup Table2/1 -> Quantizer9/1
  1-D Lookup Table1/1 -> Mux5/2  "Data"
  1-D Lookup Table3/1 -> Mux5/3

== system ADU_Integration_Y2016_simulation/LogData/Sensor_ESR/Data_4 ==
  1-D Lookup Table1 : Lookup_n-D  NumberOfTableDimensions=1  BreakpointsForDimension1=TestData_001.X.Data  Table=TestData_001.Y(206+4*a).Data  RndMeth=Simplest  InputSameDT=on
  1-D Lookup Table2 : Lookup_n-D  NumberOfTableDimensions=1  BreakpointsForDimension1=TestData_001.X.Data  Table=TestData_001.Y(205+4*a).Data  RndMeth=Simplest  InputSameDT=on
  1-D Lookup Table3 : Lookup_n-D  NumberOfTableDimensions=1  BreakpointsForDimension1=TestData_001.X.Data  Table=TestData_001.Y(207+4*a).Data  RndMeth=Simplest  InputSameDT=on
  1-D Lookup Table4 : Lookup_n-D  NumberOfTableDimensions=1  BreakpointsForDimension1=TestData_001.X.Data  Table=TestData_001.Y(208+4*a).Data  RndMeth=Simplest  InputSameDT=on
  Mux5 : Mux
  Quantizer9 : Quantizer  QuantizationInterval=1
  Out1 : Outport
  wires:
  1-D Lookup Table3/1 -> Mux5/3
  1-D Lookup Table1/1 -> Mux5/2  "Data"
  1-D Lookup Table2/1 -> Quantizer9/1
  Quantizer9/1 -> Mux5/1
  1-D Lookup Table4/1 -> Mux5/4
  [Clock] -> 1-D Lookup Table1/1, 1-D Lookup Table3/1, 1-D Lookup Table4/1, 1-D Lookup Table2/1
  Mux5/1 -> Out1/1

== system ADU_Integration_Y2016_simulation/LogData/Sensor_ESR/Data_40 ==
  1-D Lookup Table1 : Lookup_n-D  NumberOfTableDimensions=1  BreakpointsForDimension1=TestData_001.X.Data  Table=TestData_001.Y(206+4*a).Data  RndMeth=Simplest  InputSameDT=on
  1-D Lookup Table2 : Lookup_n-D  NumberOfTableDimensions=1  BreakpointsForDimension1=TestData_001.X.Data  Table=TestData_001.Y(205+4*a).Data  RndMeth=Simplest  InputSameDT=on
  1-D Lookup Table3 : Lookup_n-D  NumberOfTableDimensions=1  BreakpointsForDimension1=TestData_001.X.Data  Table=TestData_001.Y(207+4*a).Data  RndMeth=Simplest  InputSameDT=on
  1-D Lookup Table4 : Lookup_n-D  NumberOfTableDimensions=1  BreakpointsForDimension1=TestData_001.X.Data  Table=TestData_001.Y(208+4*a).Data  RndMeth=Simplest  InputSameDT=on
  Mux5 : Mux
  Quantizer9 : Quantizer  QuantizationInterval=1
  Out1 : Outport
  wires:
  1-D Lookup Table3/1 -> Mux5/3
  1-D Lookup Table1/1 -> Mux5/2  "Data"
  1-D Lookup Table2/1 -> Quantizer9/1
  Quantizer9/1 -> Mux5/1
  1-D Lookup Table4/1 -> Mux5/4
  [Clock] -> 1-D Lookup Table1/1, 1-D Lookup Table3/1, 1-D Lookup Table4/1, 1-D Lookup Table2/1
  Mux5/1 -> Out1/1

== system ADU_Integration_Y2016_simulation/LogData/Sensor_ESR/Data_41 ==
  1-D Lookup Table1 : Lookup_n-D  NumberOfTableDimensions=1  BreakpointsForDimension1=TestData_001.X.Data  Table=TestData_001.Y(206+4*a).Data  RndMeth=Simplest  InputSameDT=on
  1-D Lookup Table2 : Lookup_n-D  NumberOfTableDimensions=1  BreakpointsForDimension1=TestData_001.X.Data  Table=TestData_001.Y(205+4*a).Data  RndMeth=Simplest  InputSameDT=on
  1-D Lookup Table3 : Lookup_n-D  NumberOfTableDimensions=1  BreakpointsForDimension1=TestData_001.X.Data  Table=TestData_001.Y(207+4*a).Data  RndMeth=Simplest  InputSameDT=on
  1-D Lookup Table4 : Lookup_n-D  NumberOfTableDimensions=1  BreakpointsForDimension1=TestData_001.X.Data  Table=TestData_001.Y(208+4*a).Data  RndMeth=Simplest  InputSameDT=on
  Mux5 : Mux
  Quantizer9 : Quantizer  QuantizationInterval=1
  Out1 : Outport
  wires:
  Mux5/1 -> Out1/1
  [Clock] -> 1-D Lookup Table2/1, 1-D Lookup Table4/1, 1-D Lookup Table3/1, 1-D Lookup Table1/1
  1-D Lookup Table4/1 -> Mux5/4
  Quantizer9/1 -> Mux5/1
  1-D Lookup Table2/1 -> Quantizer9/1
  1-D Lookup Table1/1 -> Mux5/2  "Data"
  1-D Lookup Table3/1 -> Mux5/3

== system ADU_Integration_Y2016_simulation/LogData/Sensor_ESR/Data_42 ==
  1-D Lookup Table1 : Lookup_n-D  NumberOfTableDimensions=1  BreakpointsForDimension1=TestData_001.X.Data  Table=TestData_001.Y(206+4*a).Data  RndMeth=Simplest  InputSameDT=on
  1-D Lookup Table2 : Lookup_n-D  NumberOfTableDimensions=1  BreakpointsForDimension1=TestData_001.X.Data  Table=TestData_001.Y(205+4*a).Data  RndMeth=Simplest  InputSameDT=on
  1-D Lookup Table3 : Lookup_n-D  NumberOfTableDimensions=1  BreakpointsForDimension1=TestData_001.X.Data  Table=TestData_001.Y(207+4*a).Data  RndMeth=Simplest  InputSameDT=on
  1-D Lookup Table4 : Lookup_n-D  NumberOfTableDimensions=1  BreakpointsForDimension1=TestData_001.X.Data  Table=TestData_001.Y(208+4*a).Data  RndMeth=Simplest  InputSameDT=on
  Mux5 : Mux
  Quantizer9 : Quantizer  QuantizationInterval=1
  Out1 : Outport
  wires:
  1-D Lookup Table3/1 -> Mux5/3
  1-D Lookup Table1/1 -> Mux5/2  "Data"
  1-D Lookup Table2/1 -> Quantizer9/1
  Quantizer9/1 -> Mux5/1
  1-D Lookup Table4/1 -> Mux5/4
  [Clock] -> 1-D Lookup Table1/1, 1-D Lookup Table3/1, 1-D Lookup Table4/1, 1-D Lookup Table2/1
  Mux5/1 -> Out1/1

== system ADU_Integration_Y2016_simulation/LogData/Sensor_ESR/Data_43 ==
  1-D Lookup Table1 : Lookup_n-D  NumberOfTableDimensions=1  BreakpointsForDimension1=TestData_001.X.Data  Table=TestData_001.Y(206+4*a).Data  RndMeth=Simplest  InputSameDT=on
  1-D Lookup Table2 : Lookup_n-D  NumberOfTableDimensions=1  BreakpointsForDimension1=TestData_001.X.Data  Table=TestData_001.Y(205+4*a).Data  RndMeth=Simplest  InputSameDT=on
  1-D Lookup Table3 : Lookup_n-D  NumberOfTableDimensions=1  BreakpointsForDimension1=TestData_001.X.Data  Table=TestData_001.Y(207+4*a).Data  RndMeth=Simplest  InputSameDT=on
  1-D Lookup Table4 : Lookup_n-D  NumberOfTableDimensions=1  BreakpointsForDimension1=TestData_001.X.Data  Table=TestData_001.Y(208+4*a).Data  RndMeth=Simplest  InputSameDT=on
  Mux5 : Mux
  Quantizer9 : Quantizer  QuantizationInterval=1
  Out1 : Outport
  wires:
  Mux5/1 -> Out1/1
  [Clock] -> 1-D Lookup Table2/1, 1-D Lookup Table4/1, 1-D Lookup Table3/1, 1-D Lookup Table1/1
  1-D Lookup Table4/1 -> Mux5/4
  Quantizer9/1 -> Mux5/1
  1-D Lookup Table2/1 -> Quantizer9/1
  1-D Lookup Table1/1 -> Mux5/2  "Data"
  1-D Lookup Table3/1 -> Mux5/3

== system ADU_Integration_Y2016_simulation/LogData/Sensor_ESR/Data_44 ==
  1-D Lookup Table1 : Lookup_n-D  NumberOfTableDimensions=1  BreakpointsForDimension1=TestData_001.X.Data  Table=TestData_001.Y(206+4*a).Data  RndMeth=Simplest  InputSameDT=on
  1-D Lookup Table2 : Lookup_n-D  NumberOfTableDimensions=1  BreakpointsForDimension1=TestData_001.X.Data  Table=TestData_001.Y(205+4*a).Data  RndMeth=Simplest  InputSameDT=on
  1-D Lookup Table3 : Lookup_n-D  NumberOfTableDimensions=1  BreakpointsForDimension1=TestData_001.X.Data  Table=TestData_001.Y(207+4*a).Data  RndMeth=Simplest  InputSameDT=on
  1-D Lookup Table4 : Lookup_n-D  NumberOfTableDimensions=1  BreakpointsForDimension1=TestData_001.X.Data  Table=TestData_001.Y(208+4*a).Data  RndMeth=Simplest  InputSameDT=on
  Mux5 : Mux
  Quantizer9 : Quantizer  QuantizationInterval=1
  Out1 : Outport
  wires:
  1-D Lookup Table3/1 -> Mux5/3
  1-D Lookup Table1/1 -> Mux5/2  "Data"
  1-D Lookup Table2/1 -> Quantizer9/1
  Quantizer9/1 -> Mux5/1
  1-D Lookup Table4/1 -> Mux5/4
  [Clock] -> 1-D Lookup Table1/1, 1-D Lookup Table3/1, 1-D Lookup Table4/1, 1-D Lookup Table2/1
  Mux5/1 -> Out1/1

== system ADU_Integration_Y2016_simulation/LogData/Sensor_ESR/Data_45 ==
  1-D Lookup Table1 : Lookup_n-D  NumberOfTableDimensions=1  BreakpointsForDimension1=TestData_001.X.Data  Table=TestData_001.Y(206+4*a).Data  RndMeth=Simplest  InputSameDT=on
  1-D Lookup Table2 : Lookup_n-D  NumberOfTableDimensions=1  BreakpointsForDimension1=TestData_001.X.Data  Table=TestData_001.Y(205+4*a).Data  RndMeth=Simplest  InputSameDT=on
  1-D Lookup Table3 : Lookup_n-D  NumberOfTableDimensions=1  BreakpointsForDimension1=TestData_001.X.Data  Table=TestData_001.Y(207+4*a).Data  RndMeth=Simplest  InputSameDT=on
  1-D Lookup Table4 : Lookup_n-D  NumberOfTableDimensions=1  BreakpointsForDimension1=TestData_001.X.Data  Table=TestData_001.Y(208+4*a).Data  RndMeth=Simplest  InputSameDT=on
  Mux5 : Mux
  Quantizer9 : Quantizer  QuantizationInterval=1
  Out1 : Outport
  wires:
  Mux5/1 -> Out1/1
  [Clock] -> 1-D Lookup Table2/1, 1-D Lookup Table4/1, 1-D Lookup Table3/1, 1-D Lookup Table1/1
  1-D Lookup Table4/1 -> Mux5/4
  Quantizer9/1 -> Mux5/1
  1-D Lookup Table2/1 -> Quantizer9/1
  1-D Lookup Table1/1 -> Mux5/2  "Data"
  1-D Lookup Table3/1 -> Mux5/3

== system ADU_Integration_Y2016_simulation/LogData/Sensor_ESR/Data_46 ==
  1-D Lookup Table1 : Lookup_n-D  NumberOfTableDimensions=1  BreakpointsForDimension1=TestData_001.X.Data  Table=TestData_001.Y(206+4*a).Data  RndMeth=Simplest  InputSameDT=on
  1-D Lookup Table2 : Lookup_n-D  NumberOfTableDimensions=1  BreakpointsForDimension1=TestData_001.X.Data  Table=TestData_001.Y(205+4*a).Data  RndMeth=Simplest  InputSameDT=on
  1-D Lookup Table3 : Lookup_n-D  NumberOfTableDimensions=1  BreakpointsForDimension1=TestData_001.X.Data  Table=TestData_001.Y(207+4*a).Data  RndMeth=Simplest  InputSameDT=on
  1-D Lookup Table4 : Lookup_n-D  NumberOfTableDimensions=1  BreakpointsForDimension1=TestData_001.X.Data  Table=TestData_001.Y(208+4*a).Data  RndMeth=Simplest  InputSameDT=on
  Mux5 : Mux
  Quantizer9 : Quantizer  QuantizationInterval=1
  Out1 : Outport
  wires:
  1-D Lookup Table3/1 -> Mux5/3
  1-D Lookup Table1/1 -> Mux5/2  "Data"
  1-D Lookup Table2/1 -> Quantizer9/1
  Quantizer9/1 -> Mux5/1
  1-D Lookup Table4/1 -> Mux5/4
  [Clock] -> 1-D Lookup Table1/1, 1-D Lookup Table3/1, 1-D Lookup Table4/1, 1-D Lookup Table2/1
  Mux5/1 -> Out1/1

== system ADU_Integration_Y2016_simulation/LogData/Sensor_ESR/Data_47 ==
  1-D Lookup Table1 : Lookup_n-D  NumberOfTableDimensions=1  BreakpointsForDimension1=TestData_001.X.Data  Table=TestData_001.Y(206+4*a).Data  RndMeth=Simplest  InputSameDT=on
  1-D Lookup Table2 : Lookup_n-D  NumberOfTableDimensions=1  BreakpointsForDimension1=TestData_001.X.Data  Table=TestData_001.Y(205+4*a).Data  RndMeth=Simplest  InputSameDT=on
  1-D Lookup Table3 : Lookup_n-D  NumberOfTableDimensions=1  BreakpointsForDimension1=TestData_001.X.Data  Table=TestData_001.Y(207+4*a).Data  RndMeth=Simplest  InputSameDT=on
  1-D Lookup Table4 : Lookup_n-D  NumberOfTableDimensions=1  BreakpointsForDimension1=TestData_001.X.Data  Table=TestData_001.Y(208+4*a).Data  RndMeth=Simplest  InputSameDT=on
  Mux5 : Mux
  Quantizer9 : Quantizer  QuantizationInterval=1
  Out1 : Outport
  wires:
  Mux5/1 -> Out1/1
  [Clock] -> 1-D Lookup Table2/1, 1-D Lookup Table4/1, 1-D Lookup Table3/1, 1-D Lookup Table1/1
  1-D Lookup Table4/1 -> Mux5/4
  Quantizer9/1 -> Mux5/1
  1-D Lookup Table2/1 -> Quantizer9/1
  1-D Lookup Table1/1 -> Mux5/2  "Data"
  1-D Lookup Table3/1 -> Mux5/3

== system ADU_Integration_Y2016_simulation/LogData/Sensor_ESR/Data_48 ==
  1-D Lookup Table1 : Lookup_n-D  NumberOfTableDimensions=1  BreakpointsForDimension1=TestData_001.X.Data  Table=TestData_001.Y(206+4*a).Data  RndMeth=Simplest  InputSameDT=on
  1-D Lookup Table2 : Lookup_n-D  NumberOfTableDimensions=1  BreakpointsForDimension1=TestData_001.X.Data  Table=TestData_001.Y(205+4*a).Data  RndMeth=Simplest  InputSameDT=on
  1-D Lookup Table3 : Lookup_n-D  NumberOfTableDimensions=1  BreakpointsForDimension1=TestData_001.X.Data  Table=TestData_001.Y(207+4*a).Data  RndMeth=Simplest  InputSameDT=on
  1-D Lookup Table4 : Lookup_n-D  NumberOfTableDimensions=1  BreakpointsForDimension1=TestData_001.X.Data  Table=TestData_001.Y(208+4*a).Data  RndMeth=Simplest  InputSameDT=on
  Mux5 : Mux
  Quantizer9 : Quantizer  QuantizationInterval=1
  Out1 : Outport
  wires:
  1-D Lookup Table3/1 -> Mux5/3
  1-D Lookup Table1/1 -> Mux5/2  "Data"
  1-D Lookup Table2/1 -> Quantizer9/1
  Quantizer9/1 -> Mux5/1
  1-D Lookup Table4/1 -> Mux5/4
  [Clock] -> 1-D Lookup Table1/1, 1-D Lookup Table3/1, 1-D Lookup Table4/1, 1-D Lookup Table2/1
  Mux5/1 -> Out1/1

== system ADU_Integration_Y2016_simulation/LogData/Sensor_ESR/Data_49 ==
  1-D Lookup Table1 : Lookup_n-D  NumberOfTableDimensions=1  BreakpointsForDimension1=TestData_001.X.Data  Table=TestData_001.Y(206+4*a).Data  RndMeth=Simplest  InputSameDT=on
  1-D Lookup Table2 : Lookup_n-D  NumberOfTableDimensions=1  BreakpointsForDimension1=TestData_001.X.Data  Table=TestData_001.Y(205+4*a).Data  RndMeth=Simplest  InputSameDT=on
  1-D Lookup Table3 : Lookup_n-D  NumberOfTableDimensions=1  BreakpointsForDimension1=TestData_001.X.Data  Table=TestData_001.Y(207+4*a).Data  RndMeth=Simplest  InputSameDT=on
  1-D Lookup Table4 : Lookup_n-D  NumberOfTableDimensions=1  BreakpointsForDimension1=TestData_001.X.Data  Table=TestData_001.Y(208+4*a).Data  RndMeth=Simplest  InputSameDT=on
  Mux5 : Mux
  Quantizer9 : Quantizer  QuantizationInterval=1
  Out1 : Outport
  wires:
  Mux5/1 -> Out1/1
  [Clock] -> 1-D Lookup Table2/1, 1-D Lookup Table4/1, 1-D Lookup Table3/1, 1-D Lookup Table1/1
  1-D Lookup Table4/1 -> Mux5/4
  Quantizer9/1 -> Mux5/1
  1-D Lookup Table2/1 -> Quantizer9/1
  1-D Lookup Table1/1 -> Mux5/2  "Data"
  1-D Lookup Table3/1 -> Mux5/3

== system ADU_Integration_Y2016_simulation/LogData/Sensor_ESR/Data_5 ==
  1-D Lookup Table1 : Lookup_n-D  NumberOfTableDimensions=1  BreakpointsForDimension1=TestData_001.X.Data  Table=TestData_001.Y(206+4*a).Data  RndMeth=Simplest  InputSameDT=on
  1-D Lookup Table2 : Lookup_n-D  NumberOfTableDimensions=1  BreakpointsForDimension1=TestData_001.X.Data  Table=TestData_001.Y(205+4*a).Data  RndMeth=Simplest  InputSameDT=on
  1-D Lookup Table3 : Lookup_n-D  NumberOfTableDimensions=1  BreakpointsForDimension1=TestData_001.X.Data  Table=TestData_001.Y(207+4*a).Data  RndMeth=Simplest  InputSameDT=on
  1-D Lookup Table4 : Lookup_n-D  NumberOfTableDimensions=1  BreakpointsForDimension1=TestData_001.X.Data  Table=TestData_001.Y(208+4*a).Data  RndMeth=Simplest  InputSameDT=on
  Mux5 : Mux
  Quantizer9 : Quantizer  QuantizationInterval=1
  Out1 : Outport
  wires:
  Mux5/1 -> Out1/1
  [Clock] -> 1-D Lookup Table2/1, 1-D Lookup Table4/1, 1-D Lookup Table3/1, 1-D Lookup Table1/1
  1-D Lookup Table4/1 -> Mux5/4
  Quantizer9/1 -> Mux5/1
  1-D Lookup Table2/1 -> Quantizer9/1
  1-D Lookup Table1/1 -> Mux5/2  "Data"
  1-D Lookup Table3/1 -> Mux5/3

== system ADU_Integration_Y2016_simulation/LogData/Sensor_ESR/Data_50 ==
  1-D Lookup Table1 : Lookup_n-D  NumberOfTableDimensions=1  BreakpointsForDimension1=TestData_001.X.Data  Table=TestData_001.Y(206+4*a).Data  RndMeth=Simplest  InputSameDT=on
  1-D Lookup Table2 : Lookup_n-D  NumberOfTableDimensions=1  BreakpointsForDimension1=TestData_001.X.Data  Table=TestData_001.Y(205+4*a).Data  RndMeth=Simplest  InputSameDT=on
  1-D Lookup Table3 : Lookup_n-D  NumberOfTableDimensions=1  BreakpointsForDimension1=TestData_001.X.Data  Table=TestData_001.Y(207+4*a).Data  RndMeth=Simplest  InputSameDT=on
  1-D Lookup Table4 : Lookup_n-D  NumberOfTableDimensions=1  BreakpointsForDimension1=TestData_001.X.Data  Table=TestData_001.Y(208+4*a).Data  RndMeth=Simplest  InputSameDT=on
  Mux5 : Mux
  Quantizer9 : Quantizer  QuantizationInterval=1
  Out1 : Outport
  wires:
  1-D Lookup Table3/1 -> Mux5/3
  1-D Lookup Table1/1 -> Mux5/2  "Data"
  1-D Lookup Table2/1 -> Quantizer9/1
  Quantizer9/1 -> Mux5/1
  1-D Lookup Table4/1 -> Mux5/4
  [Clock] -> 1-D Lookup Table1/1, 1-D Lookup Table3/1, 1-D Lookup Table4/1, 1-D Lookup Table2/1
  Mux5/1 -> Out1/1
